simulink model "Transitions3"  (R2020a)
settings: Solver=VariableStepAuto  StartTime=0.0  StopTime=0.5  RelTol=1e-3
settings Model: Creator=86188  LastModifiedBy=bzhan
settings DataIOCC: ReturnWorkspaceOutputs=off
settings DebuggingCC: ArithmeticOperatorsInVariantConditions=warning
settings SFSimCC: SimUseLocalCustomCode=off  CustomCodeUndefinedFunction=UseInterfaceOnly
settings RTWCC: RTWUseLocalCustomCode=off

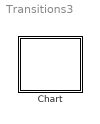
== system Transitions3 ==
  Chart : Stateflow chart  TreatAsAtomicUnit=on

== stateflow chart Transitions3/Chart ==
  settings: updateMethod=DISCRETE  sampleTime=0.1
  state A
    (history)
    state b
      en: f("b")
    state c
      (history)
      state c1
        en: f("c1")
      state c2
        en: f("c2")
      (default) -> c1
      c1 -> c2
    (default) -> b
    b -> c
  state B
    en: f("B")
  (default) -> A
  B -> A
  c2 -> B
  data: s function_input
  function f(s):
    | function f(s)
    |   fprintf(s+"\n");
